simulink model "PI_controller"  (R2018a)
settings: Solver=VariableStepAuto  StartTime=0.0  StopTime=120  RelTol=1e-3
settings Model: Creator=mjb15180  LastModifiedBy=mjb15180

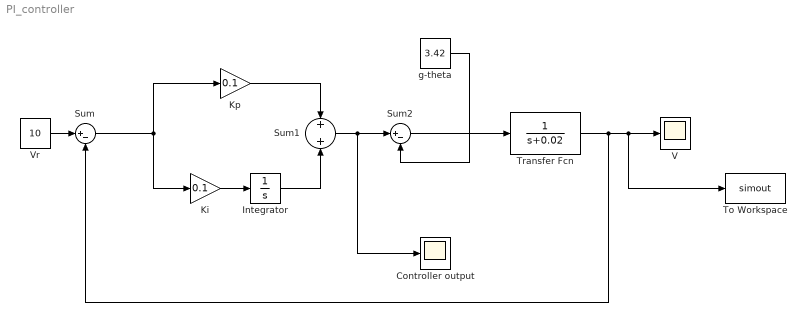
== system PI_controller ==
  Controller output : Scope
  Integrator : Integrator  InitialCondition=1
  Ki : Gain  Gain=0.1
  Kp : Gain  Gain=0.1
  Sum : Sum  Inputs=|+-
  Sum1 : Sum
  Sum2 : Sum  Inputs=|+-
  To Workspace : ToWorkspace  VariableName=simout  SaveFormat=Timeseries  SampleTime=-1
  Transfer Fcn : TransferFcn  Denominator=[1 0.02]
  V : Scope
  Vr : Constant  Value=10
  g-theta : Constant  Value=3.42
  wires:
  Sum/1 -> Kp/1, Ki/1
  Ki/1 -> Integrator/1
  Integrator/1 -> Sum1/2
  Kp/1 -> Sum1/1
  Sum1/1 -> Controller output/1, Sum2/1
  g-theta/1 -> Sum2/2
  Sum2/1 -> Transfer Fcn/1
  Transfer Fcn/1 -> To Workspace/1, V/1, Sum/2
  Vr/1 -> Sum/1
